simulink model "SystemComposer_Architecture"  (R2020a)
settings: Solver=VariableStepAuto  StartTime=0.0  StopTime=10.0  RelTol=1e-3
settings Model: Creator=pav4609  LastModifiedBy=pav4609

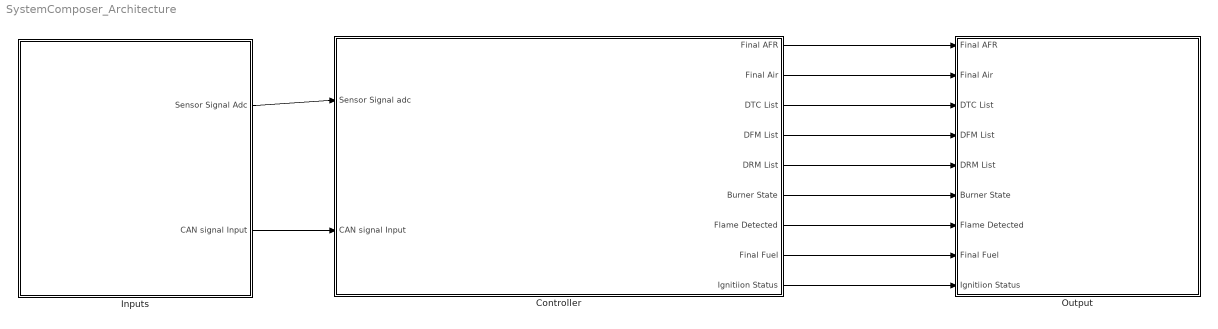
== system SystemComposer_Architecture ==
  Controller : Subsystem
      settings: PortSchema="{\"entries\":[{\"content\":{\"headerSize\":26,\"margin\":15,\"minimumSpacing\":25,\"sides\":[{\"content\":{\"connectorIds\":[\"In1\",\"In2\"]},\"type\":\"ConnectorPlacement.EquallySpacedRectSide\",\"uuid\":\"096bda3c-cb26-41de-ada6-ed8c82f4dc3e\"},{\"content\":{\"connectorIds\":[\"Out1\",\"Out2\",\"Out3\",\"Out4\",\"Out5\",\"Out6\",\"Out7\",\"Out8\",\"Out9\"],\"side\":\"RIGHT\"},\"type\":\"ConnectorPlacement.EquallySpacedRectSide\",\"uuid\":\"33a8afe9-c0b7-4d1e-b92f-6038b85d7ed2\"},{\"content\":{\"connectorIds\":[],\"side\":\"TOP\"},\"type\":\"ConnectorPlacement.EquallySpacedRectSide\",\"uuid\":\"f728da00-d767-486c-a498-31860175d68d\"}]},\"type\":\"ConnectorPlacement.EquallySpacedConnector\",\"uuid\":\"b1077154-7336-4249-93d2-0c64e27b627c\"}],\"packageUris\":[\"http://schema.mathworks.com/mf0/Connector/19700101\"],\"version\":\"1.0\"}"
  Inputs : Subsystem
      settings: PortSchema="{\"entries\":[{\"content\":{\"headerSize\":26,\"margin\":15,\"minimumSpacing\":25,\"sides\":[{\"content\":{\"connectorIds\":[]},\"type\":\"ConnectorPlacement.EquallySpacedRectSide\",\"uuid\":\"096bda3c-cb26-41de-ada6-ed8c82f4dc3e\"},{\"content\":{\"connectorIds\":[\"Out1\",\"Out2\"],\"side\":\"RIGHT\"},\"type\":\"ConnectorPlacement.EquallySpacedRectSide\",\"uuid\":\"33a8afe9-c0b7-4d1e-b92f-6038b85d7ed2\"},{\"content\":{\"connectorIds\":[],\"side\":\"TOP\"},\"type\":\"ConnectorPlacement.EquallySpacedRectSide\",\"uuid\":\"f728da00-d767-486c-a498-31860175d68d\"}]},\"type\":\"ConnectorPlacement.EquallySpacedConnector\",\"uuid\":\"b1077154-7336-4249-93d2-0c64e27b627c\"}],\"packageUris\":[\"http://schema.mathworks.com/mf0/Connector/19700101\"],\"version\":\"1.0\"}"
  Output : Subsystem
      settings: PortSchema="{\"entries\":[{\"content\":{\"headerSize\":26,\"margin\":15,\"minimumSpacing\":25,\"sides\":[{\"content\":{\"connectorIds\":[\"In3\",\"In4\",\"In5\",\"In6\",\"In7\",\"In8\",\"In9\",\"In1\",\"In2\"]},\"type\":\"ConnectorPlacement.EquallySpacedRectSide\",\"uuid\":\"096bda3c-cb26-41de-ada6-ed8c82f4dc3e\"},{\"content\":{\"connectorIds\":[],\"side\":\"RIGHT\"},\"type\":\"ConnectorPlacement.EquallySpacedRectSide\",\"uuid\":\"33a8afe9-c0b7-4d1e-b92f-6038b85d7ed2\"},{\"content\":{\"connectorIds\":[],\"side\":\"TOP\"},\"type\":\"ConnectorPlacement.EquallySpacedRectSide\",\"uuid\":\"f728da00-d767-486c-a498-31860175d68d\"},{\"content\":{\"connectorIds\":[],\"side\":\"BOTTOM\"},\"type\":\"ConnectorPlacement.EquallySpacedRectSide\",\"uuid\":\"2b26c1e7-6ba1-4f96-9e0c-c596cf4da347\"}]},\"type\":\"ConnectorPlacement.EquallySpacedConnector\",\"uuid\":\"b1077154-7336-4249-93d2-0c64e27b627c\"}],\"packageUris\":[\"http://schema.mathworks.com/mf0/Connector/19700101\"],\"version\":\"1.0\"}"
  wires:
  Inputs/1(Sensor Signal Adc) -> Controller/1(Sensor Signal adc)
  Inputs/2(CAN signal Input) -> Controller/2(CAN signal Input)
  Controller/1(Final AFR) -> Output/3(Final AFR)
  Controller/2(Final Air) -> Output/4(Final Air)
  Controller/3(DTC List) -> Output/5(DTC List)
  Controller/4(DFM List) -> Output/6(DFM List)
  Controller/5(DRM List) -> Output/7(DRM List)
  Controller/6(Burner State) -> Output/8(Burner State)
  Controller/7(Flame Detected) -> Output/9(Flame Detected)
  Controller/8(Final Fuel) -> Output/1(Final Fuel)
  Controller/9(Ignitiion Status) -> Output/2(Ignitiion Status)

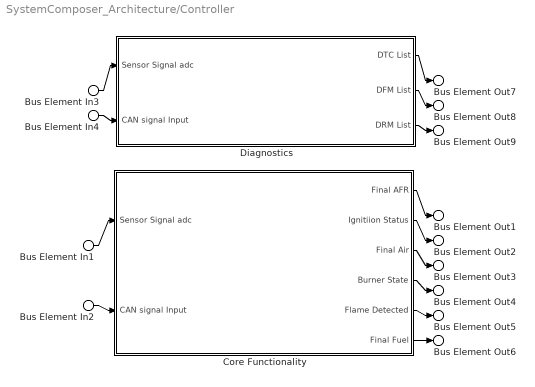
== system SystemComposer_Architecture/Controller ==
  Bus Element In1 : Inport  PortName=Sensor Signal adc
  Bus Element In3 : Inport  PortName=Sensor Signal adc
  Bus Element In2 : Inport  Port=2  PortName=CAN signal Input
  Bus Element In4 : Inport  Port=2  PortName=CAN signal Input
  Core Functionality : Subsystem
      settings: PortSchema="{\"entries\":[{\"content\":{\"headerSize\":26,\"margin\":15,\"minimumSpacing\":25,\"sides\":[{\"content\":{\"connectorIds\":[\"In1\",\"In2\"]},\"type\":\"ConnectorPlacement.EquallySpacedRectSide\",\"uuid\":\"096bda3c-cb26-41de-ada6-ed8c82f4dc3e\"},{\"content\":{\"connectorIds\":[\"Out1\",\"Out2\",\"Out3\",\"Out4\",\"Out5\",\"Out6\"],\"side\":\"RIGHT\"},\"type\":\"ConnectorPlacement.EquallySpacedRectSide\",\"uuid\":\"33a8afe9-c0b7-4d1e-b92f-6038b85d7ed2\"},{\"content\":{\"connectorIds\":[],\"side\":\"TOP\"},\"type\":\"ConnectorPlacement.EquallySpacedRectSide\",\"uuid\":\"f728da00-d767-486c-a498-31860175d68d\"}]},\"type\":\"ConnectorPlacement.EquallySpacedConnector\",\"uuid\":\"b1077154-7336-4249-93d2-0c64e27b627c\"}],\"packageUris\":[\"http://schema.mathworks.com/mf0/Connector/19700101\"],\"version\":\"1.0\"}"
  Diagnostics : Subsystem
      settings: PortSchema="{\"entries\":[{\"content\":{\"headerSize\":26,\"margin\":15,\"minimumSpacing\":25,\"sides\":[{\"content\":{\"connectorIds\":[\"In1\",\"In2\"]},\"type\":\"ConnectorPlacement.EquallySpacedRectSide\",\"uuid\":\"096bda3c-cb26-41de-ada6-ed8c82f4dc3e\"},{\"content\":{\"connectorIds\":[\"Out1\",\"Out2\",\"Out3\"],\"side\":\"RIGHT\"},\"type\":\"ConnectorPlacement.EquallySpacedRectSide\",\"uuid\":\"33a8afe9-c0b7-4d1e-b92f-6038b85d7ed2\"},{\"content\":{\"connectorIds\":[],\"side\":\"TOP\"},\"type\":\"ConnectorPlacement.EquallySpacedRectSide\",\"uuid\":\"f728da00-d767-486c-a498-31860175d68d\"}]},\"type\":\"ConnectorPlacement.EquallySpacedConnector\",\"uuid\":\"b1077154-7336-4249-93d2-0c64e27b627c\"}],\"packageUris\":[\"http://schema.mathworks.com/mf0/Connector/19700101\"],\"version\":\"1.0\"}"
  Bus Element Out1 : Outport  PortName=Final AFR
  Bus Element Out3 : Outport  Port=2  PortName=Final Air
  Bus Element Out7 : Outport  Port=3  PortName=DTC List
  Bus Element Out8 : Outport  Port=4  PortName=DFM List
  Bus Element Out9 : Outport  Port=5  PortName=DRM List
  Bus Element Out4 : Outport  Port=6  PortName=Burner State
  Bus Element Out5 : Outport  Port=7  PortName=Flame Detected
  Bus Element Out6 : Outport  Port=8  PortName=Final Fuel
  Bus Element Out2 : Outport  Port=9  PortName=Ignitiion Status
  wires:
  Bus Element In1/1 -> Core Functionality/1(Sensor Signal adc)
  Bus Element In2/1 -> Core Functionality/2(CAN signal Input)
  Bus Element In3/1 -> Diagnostics/1(Sensor Signal adc)
  Bus Element In4/1 -> Diagnostics/2(CAN signal Input)
  Core Functionality/1(Final AFR) -> Bus Element Out1/1
  Core Functionality/2(Ignitiion Status) -> Bus Element Out2/1
  Core Functionality/3(Final Air) -> Bus Element Out3/1
  Core Functionality/4(Burner State) -> Bus Element Out4/1
  Core Functionality/5(Flame Detected) -> Bus Element Out5/1
  Core Functionality/6(Final Fuel) -> Bus Element Out6/1
  Diagnostics/1(DTC List) -> Bus Element Out7/1
  Diagnostics/2(DFM List) -> Bus Element Out8/1
  Diagnostics/3(DRM List) -> Bus Element Out9/1

== system SystemComposer_Architecture/Inputs ==
  CAN : Subsystem
      settings: PortSchema="{\"entries\":[{\"content\":{\"headerSize\":26,\"margin\":15,\"minimumSpacing\":25,\"sides\":[{\"content\":{\"connectorIds\":[]},\"type\":\"ConnectorPlacement.EquallySpacedRectSide\",\"uuid\":\"096bda3c-cb26-41de-ada6-ed8c82f4dc3e\"},{\"content\":{\"connectorIds\":[\"Out1\"],\"side\":\"RIGHT\"},\"type\":\"ConnectorPlacement.EquallySpacedRectSide\",\"uuid\":\"33a8afe9-c0b7-4d1e-b92f-6038b85d7ed2\"},{\"content\":{\"connectorIds\":[],\"side\":\"TOP\"},\"type\":\"ConnectorPlacement.EquallySpacedRectSide\",\"uuid\":\"f728da00-d767-486c-a498-31860175d68d\"}]},\"type\":\"ConnectorPlacement.EquallySpacedConnector\",\"uuid\":\"b1077154-7336-4249-93d2-0c64e27b627c\"}],\"packageUris\":[\"http://schema.mathworks.com/mf0/Connector/19700101\"],\"version\":\"1.0\"}"
  Sensors : Subsystem
      settings: PortSchema="{\"entries\":[{\"content\":{\"headerSize\":26,\"margin\":15,\"minimumSpacing\":25,\"sides\":[{\"content\":{\"connectorIds\":[]},\"type\":\"ConnectorPlacement.EquallySpacedRectSide\",\"uuid\":\"096bda3c-cb26-41de-ada6-ed8c82f4dc3e\"},{\"content\":{\"connectorIds\":[\"Out1\"],\"side\":\"RIGHT\"},\"type\":\"ConnectorPlacement.EquallySpacedRectSide\",\"uuid\":\"33a8afe9-c0b7-4d1e-b92f-6038b85d7ed2\"},{\"content\":{\"connectorIds\":[],\"side\":\"TOP\"},\"type\":\"ConnectorPlacement.EquallySpacedRectSide\",\"uuid\":\"f728da00-d767-486c-a498-31860175d68d\"}]},\"type\":\"ConnectorPlacement.EquallySpacedConnector\",\"uuid\":\"b1077154-7336-4249-93d2-0c64e27b627c\"}],\"packageUris\":[\"http://schema.mathworks.com/mf0/Connector/19700101\"],\"version\":\"1.0\"}"
  Bus Element Out1 : Outport  PortName=Sensor Signal Adc
  Bus Element Out2 : Outport  Port=2  PortName=CAN signal Input
  wires:
  Sensors/1(Sensor Signal Adc) -> Bus Element Out1/1
  CAN/1(CAN signal Input) -> Bus Element Out2/1

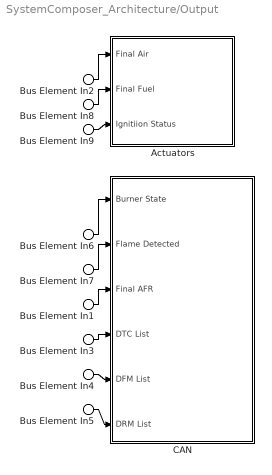
== system SystemComposer_Architecture/Output ==
  Bus Element In8 : Inport  PortName=Final Fuel
  Bus Element In9 : Inport  Port=2  PortName=Ignitiion Status
  Bus Element In1 : Inport  Port=3  PortName=Final AFR
  Bus Element In2 : Inport  Port=4  PortName=Final Air
  Bus Element In3 : Inport  Port=5  PortName=DTC List
  Bus Element In4 : Inport  Port=6  PortName=DFM List
  Bus Element In5 : Inport  Port=7  PortName=DRM List
  Bus Element In6 : Inport  Port=8  PortName=Burner State
  Bus Element In7 : Inport  Port=9  PortName=Flame Detected
  Actuators : Subsystem
      settings: PortSchema="{\"entries\":[{\"content\":{\"headerSize\":26,\"margin\":15,\"minimumSpacing\":25,\"sides\":[{\"content\":{\"connectorIds\":[\"In1\",\"In2\",\"In3\"]},\"type\":\"ConnectorPlacement.EquallySpacedRectSide\",\"uuid\":\"096bda3c-cb26-41de-ada6-ed8c82f4dc3e\"},{\"content\":{\"connectorIds\":[],\"side\":\"RIGHT\"},\"type\":\"ConnectorPlacement.EquallySpacedRectSide\",\"uuid\":\"33a8afe9-c0b7-4d1e-b92f-6038b85d7ed2\"},{\"content\":{\"connectorIds\":[],\"side\":\"TOP\"},\"type\":\"ConnectorPlacement.EquallySpacedRectSide\",\"uuid\":\"f728da00-d767-486c-a498-31860175d68d\"}]},\"type\":\"ConnectorPlacement.EquallySpacedConnector\",\"uuid\":\"b1077154-7336-4249-93d2-0c64e27b627c\"}],\"packageUris\":[\"http://schema.mathworks.com/mf0/Connector/19700101\"],\"version\":\"1.0\"}"
  CAN : Subsystem
      settings: PortSchema="{\"entries\":[{\"content\":{\"headerSize\":26,\"margin\":15,\"minimumSpacing\":25,\"sides\":[{\"content\":{\"connectorIds\":[\"In1\",\"In2\",\"In3\",\"In4\",\"In5\",\"In6\"]},\"type\":\"ConnectorPlacement.EquallySpacedRectSide\",\"uuid\":\"096bda3c-cb26-41de-ada6-ed8c82f4dc3e\"},{\"content\":{\"connectorIds\":[],\"side\":\"RIGHT\"},\"type\":\"ConnectorPlacement.EquallySpacedRectSide\",\"uuid\":\"33a8afe9-c0b7-4d1e-b92f-6038b85d7ed2\"},{\"content\":{\"connectorIds\":[],\"side\":\"TOP\"},\"type\":\"ConnectorPlacement.EquallySpacedRectSide\",\"uuid\":\"f728da00-d767-486c-a498-31860175d68d\"}]},\"type\":\"ConnectorPlacement.EquallySpacedConnector\",\"uuid\":\"b1077154-7336-4249-93d2-0c64e27b627c\"}],\"packageUris\":[\"http://schema.mathworks.com/mf0/Connector/19700101\"],\"version\":\"1.0\"}"
  wires:
  Bus Element In2/1 -> Actuators/1(Final Air)
  Bus Element In8/1 -> Actuators/2(Final Fuel)
  Bus Element In9/1 -> Actuators/3(Ignitiion Status)
  Bus Element In6/1 -> CAN/1(Burner State)
  Bus Element In7/1 -> CAN/2(Flame Detected)
  Bus Element In1/1 -> CAN/3(Final AFR)
  Bus Element In3/1 -> CAN/4(DTC List)
  Bus Element In4/1 -> CAN/5(DFM List)
  Bus Element In5/1 -> CAN/6(DRM List)

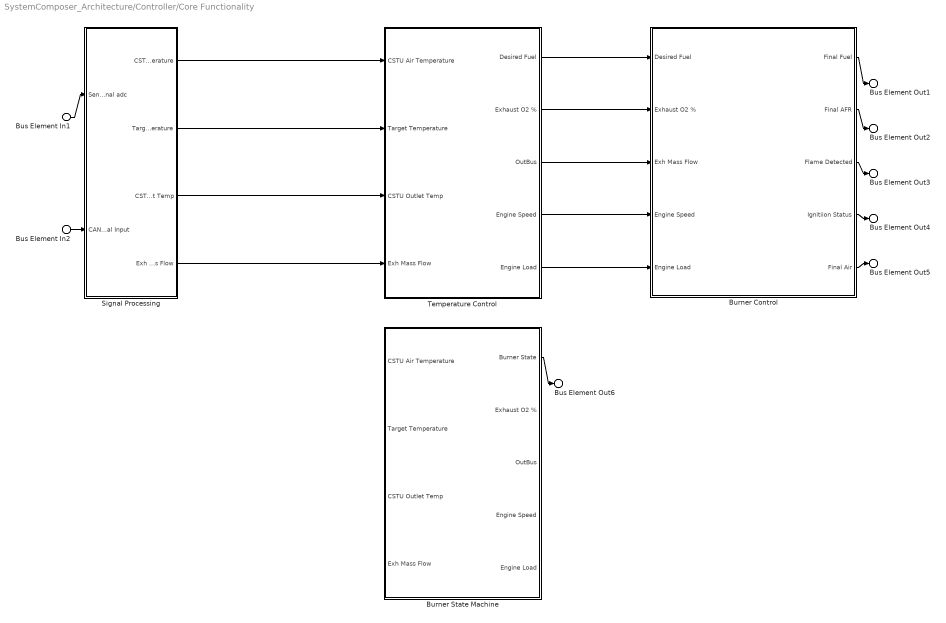
== system SystemComposer_Architecture/Controller/Core Functionality ==
  Bus Element In1 : Inport  PortName=Sensor Signal adc
  Bus Element In2 : Inport  Port=2  PortName=CAN signal Input
  Burner Control : Subsystem
      settings: PortSchema="{\"entries\":[{\"content\":{\"headerSize\":26,\"margin\":15,\"minimumSpacing\":25,\"sides\":[{\"content\":{\"connectorIds\":[\"In1\",\"In2\",\"In3\",\"In4\",\"In5\"]},\"type\":\"ConnectorPlacement.EquallySpacedRectSide\",\"uuid\":\"096bda3c-cb26-41de-ada6-ed8c82f4dc3e\"},{\"content\":{\"connectorIds\":[\"Out1\",\"Out2\",\"Out3\",\"Out4\",\"Out5\"],\"side\":\"RIGHT\"},\"type\":\"ConnectorPlacement.EquallySpacedRectSide\",\"uuid\":\"33a8afe9-c0b7-4d1e-b92f-6038b85d7ed2\"},{\"content\":{\"connectorIds\":[],\"side\":\"TOP\"},\"type\":\"ConnectorPlacement.EquallySpacedRectSide\",\"uuid\":\"f728da00-d767-486c-a498-31860175d68d\"}]},\"type\":\"ConnectorPlacement.EquallySpacedConnector\",\"uuid\":\"b1077154-7336-4249-93d2-0c64e27b627c\"}],\"packageUris\":[\"http://schema.mathworks.com/mf0/Connector/19700101\"],\"version\":\"1.0\"}"
  Burner State Machine : Subsystem
      settings: PortSchema="{\"entries\":[{\"content\":{\"headerSize\":26,\"margin\":15,\"minimumSpacing\":25,\"sides\":[{\"content\":{\"connectorIds\":[\"In1\",\"In2\",\"In3\",\"In4\"]},\"type\":\"ConnectorPlacement.EquallySpacedRectSide\",\"uuid\":\"096bda3c-cb26-41de-ada6-ed8c82f4dc3e\"},{\"content\":{\"connectorIds\":[\"Out1\",\"Out2\",\"Out3\",\"Out4\",\"Out5\"],\"side\":\"RIGHT\"},\"type\":\"ConnectorPlacement.EquallySpacedRectSide\",\"uuid\":\"33a8afe9-c0b7-4d1e-b92f-6038b85d7ed2\"},{\"content\":{\"connectorIds\":[],\"side\":\"TOP\"},\"type\":\"ConnectorPlacement.EquallySpacedRectSide\",\"uuid\":\"f728da00-d767-486c-a498-31860175d68d\"}]},\"type\":\"ConnectorPlacement.EquallySpacedConnector\",\"uuid\":\"b1077154-7336-4249-93d2-0c64e27b627c\"}],\"packageUris\":[\"http://schema.mathworks.com/mf0/Connector/19700101\"],\"version\":\"1.0\"}"
  Signal Processing : Subsystem
      settings: PortSchema="{\"entries\":[{\"content\":{\"headerSize\":26,\"margin\":15,\"minimumSpacing\":25,\"sides\":[{\"content\":{\"connectorIds\":[\"In1\",\"In2\"]},\"type\":\"ConnectorPlacement.EquallySpacedRectSide\",\"uuid\":\"096bda3c-cb26-41de-ada6-ed8c82f4dc3e\"},{\"content\":{\"connectorIds\":[\"Out1\",\"Out2\",\"Out3\",\"Out4\"],\"side\":\"RIGHT\"},\"type\":\"ConnectorPlacement.EquallySpacedRectSide\",\"uuid\":\"33a8afe9-c0b7-4d1e-b92f-6038b85d7ed2\"},{\"content\":{\"connectorIds\":[],\"side\":\"TOP\"},\"type\":\"ConnectorPlacement.EquallySpacedRectSide\",\"uuid\":\"f728da00-d767-486c-a498-31860175d68d\"}]},\"type\":\"ConnectorPlacement.EquallySpacedConnector\",\"uuid\":\"b1077154-7336-4249-93d2-0c64e27b627c\"}],\"packageUris\":[\"http://schema.mathworks.com/mf0/Connector/19700101\"],\"version\":\"1.0\"}"
  Temperature Control : Subsystem
      settings: PortSchema="{\"entries\":[{\"content\":{\"headerSize\":26,\"margin\":15,\"minimumSpacing\":25,\"sides\":[{\"content\":{\"connectorIds\":[\"In1\",\"In2\",\"In3\",\"In4\"]},\"type\":\"ConnectorPlacement.EquallySpacedRectSide\",\"uuid\":\"096bda3c-cb26-41de-ada6-ed8c82f4dc3e\"},{\"content\":{\"connectorIds\":[\"Out1\",\"Out2\",\"Out3\",\"Out4\",\"Out5\"],\"side\":\"RIGHT\"},\"type\":\"ConnectorPlacement.EquallySpacedRectSide\",\"uuid\":\"33a8afe9-c0b7-4d1e-b92f-6038b85d7ed2\"},{\"content\":{\"connectorIds\":[],\"side\":\"TOP\"},\"type\":\"ConnectorPlacement.EquallySpacedRectSide\",\"uuid\":\"f728da00-d767-486c-a498-31860175d68d\"}]},\"type\":\"ConnectorPlacement.EquallySpacedConnector\",\"uuid\":\"b1077154-7336-4249-93d2-0c64e27b627c\"}],\"packageUris\":[\"http://schema.mathworks.com/mf0/Connector/19700101\"],\"version\":\"1.0\"}"
  Bus Element Out2 : Outport  PortName=Final AFR
  Bus Element Out4 : Outport  Port=2  PortName=Ignitiion Status
  Bus Element Out5 : Outport  Port=3  PortName=Final Air
  Bus Element Out6 : Outport  Port=4  PortName=Burner State
  Bus Element Out3 : Outport  Port=5  PortName=Flame Detected
  Bus Element Out1 : Outport  Port=6  PortName=Final Fuel
  wires:
  Bus Element In1/1 -> Signal Processing/1(Sensor Signal adc)
  Bus Element In2/1 -> Signal Processing/2(CAN signal Input)
  Temperature Control/1(Desired Fuel) -> Burner Control/1(Desired Fuel)
  Temperature Control/2(Exhaust O2 %) -> Burner Control/2(Exhaust O2 %)
  Temperature Control/3(OutBus) -> Burner Control/3(Exh Mass Flow)
  Temperature Control/4(Engine Speed) -> Burner Control/4(Engine Speed)
  Temperature Control/5(Engine Load) -> Burner Control/5(Engine Load)
  Signal Processing/1(CSTU Air Temperature) -> Temperature Control/1(CSTU Air Temperature)
  Signal Processing/2(Target Temperature) -> Temperature Control/2(Target Temperature)
  Signal Processing/3(CSTU Outlet Temp) -> Temperature Control/3(CSTU Outlet Temp)
  Signal Processing/4(Exh Mass Flow) -> Temperature Control/4(Exh Mass Flow)
  Burner Control/1(Final Fuel) -> Bus Element Out1/1
  Burner Control/2(Final AFR) -> Bus Element Out2/1
  Burner Control/3(Flame Detected) -> Bus Element Out3/1
  Burner Control/4(Ignitiion Status) -> Bus Element Out4/1
  Burner Control/5(Final Air) -> Bus Element Out5/1
  Burner State Machine/1(Burner State) -> Bus Element Out6/1

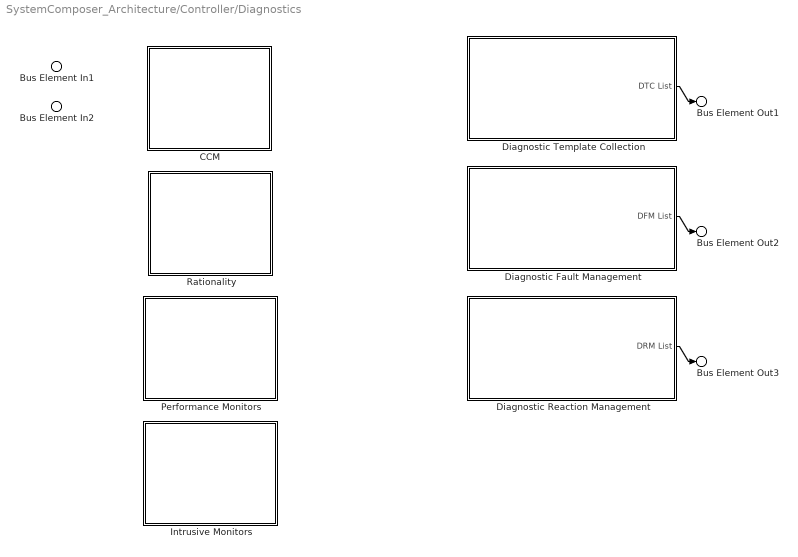
== system SystemComposer_Architecture/Controller/Diagnostics ==
  Bus Element In1 : Inport  PortName=Sensor Signal adc
  Bus Element In2 : Inport  Port=2  PortName=CAN signal Input
  CCM : Subsystem
      settings: PortSchema="{\"entries\":[{\"content\":{\"headerSize\":26,\"margin\":15,\"minimumSpacing\":25,\"sides\":[{\"content\":{\"connectorIds\":[]},\"type\":\"ConnectorPlacement.EquallySpacedRectSide\",\"uuid\":\"096bda3c-cb26-41de-ada6-ed8c82f4dc3e\"},{\"content\":{\"connectorIds\":[],\"side\":\"RIGHT\"},\"type\":\"ConnectorPlacement.EquallySpacedRectSide\",\"uuid\":\"33a8afe9-c0b7-4d1e-b92f-6038b85d7ed2\"},{\"content\":{\"connectorIds\":[],\"side\":\"TOP\"},\"type\":\"ConnectorPlacement.EquallySpacedRectSide\",\"uuid\":\"f728da00-d767-486c-a498-31860175d68d\"}]},\"type\":\"ConnectorPlacement.EquallySpacedConnector\",\"uuid\":\"b1077154-7336-4249-93d2-0c64e27b627c\"}],\"packageUris\":[\"http://schema.mathworks.com/mf0/Connector/19700101\"],\"version\":\"1.0\"}"
  Diagnostic Fault Management : Subsystem
      settings: PortSchema="{\"entries\":[{\"content\":{\"headerSize\":26,\"margin\":15,\"minimumSpacing\":25,\"sides\":[{\"content\":{\"connectorIds\":[]},\"type\":\"ConnectorPlacement.EquallySpacedRectSide\",\"uuid\":\"096bda3c-cb26-41de-ada6-ed8c82f4dc3e\"},{\"content\":{\"connectorIds\":[\"Out1\"],\"side\":\"RIGHT\"},\"type\":\"ConnectorPlacement.EquallySpacedRectSide\",\"uuid\":\"33a8afe9-c0b7-4d1e-b92f-6038b85d7ed2\"},{\"content\":{\"connectorIds\":[],\"side\":\"TOP\"},\"type\":\"ConnectorPlacement.EquallySpacedRectSide\",\"uuid\":\"f728da00-d767-486c-a498-31860175d68d\"}]},\"type\":\"ConnectorPlacement.EquallySpacedConnector\",\"uuid\":\"b1077154-7336-4249-93d2-0c64e27b627c\"}],\"packageUris\":[\"http://schema.mathworks.com/mf0/Connector/19700101\"],\"version\":\"1.0\"}"
  Diagnostic Reaction Management : Subsystem
      settings: PortSchema="{\"entries\":[{\"content\":{\"headerSize\":26,\"margin\":15,\"minimumSpacing\":25,\"sides\":[{\"content\":{\"connectorIds\":[]},\"type\":\"ConnectorPlacement.EquallySpacedRectSide\",\"uuid\":\"096bda3c-cb26-41de-ada6-ed8c82f4dc3e\"},{\"content\":{\"connectorIds\":[\"Out1\"],\"side\":\"RIGHT\"},\"type\":\"ConnectorPlacement.EquallySpacedRectSide\",\"uuid\":\"33a8afe9-c0b7-4d1e-b92f-6038b85d7ed2\"},{\"content\":{\"connectorIds\":[],\"side\":\"TOP\"},\"type\":\"ConnectorPlacement.EquallySpacedRectSide\",\"uuid\":\"f728da00-d767-486c-a498-31860175d68d\"}]},\"type\":\"ConnectorPlacement.EquallySpacedConnector\",\"uuid\":\"b1077154-7336-4249-93d2-0c64e27b627c\"}],\"packageUris\":[\"http://schema.mathworks.com/mf0/Connector/19700101\"],\"version\":\"1.0\"}"
  Diagnostic Template Collection : Subsystem
      settings: PortSchema="{\"entries\":[{\"content\":{\"headerSize\":26,\"margin\":15,\"minimumSpacing\":25,\"sides\":[{\"content\":{\"connectorIds\":[]},\"type\":\"ConnectorPlacement.EquallySpacedRectSide\",\"uuid\":\"096bda3c-cb26-41de-ada6-ed8c82f4dc3e\"},{\"content\":{\"connectorIds\":[\"Out1\"],\"side\":\"RIGHT\"},\"type\":\"ConnectorPlacement.EquallySpacedRectSide\",\"uuid\":\"33a8afe9-c0b7-4d1e-b92f-6038b85d7ed2\"},{\"content\":{\"connectorIds\":[],\"side\":\"TOP\"},\"type\":\"ConnectorPlacement.EquallySpacedRectSide\",\"uuid\":\"f728da00-d767-486c-a498-31860175d68d\"}]},\"type\":\"ConnectorPlacement.EquallySpacedConnector\",\"uuid\":\"b1077154-7336-4249-93d2-0c64e27b627c\"}],\"packageUris\":[\"http://schema.mathworks.com/mf0/Connector/19700101\"],\"version\":\"1.0\"}"
  Intrusive Monitors : Subsystem
      settings: PortSchema="{\"entries\":[{\"content\":{\"headerSize\":26,\"margin\":15,\"minimumSpacing\":25,\"sides\":[{\"content\":{\"connectorIds\":[]},\"type\":\"ConnectorPlacement.EquallySpacedRectSide\",\"uuid\":\"096bda3c-cb26-41de-ada6-ed8c82f4dc3e\"},{\"content\":{\"connectorIds\":[],\"side\":\"RIGHT\"},\"type\":\"ConnectorPlacement.EquallySpacedRectSide\",\"uuid\":\"33a8afe9-c0b7-4d1e-b92f-6038b85d7ed2\"},{\"content\":{\"connectorIds\":[],\"side\":\"TOP\"},\"type\":\"ConnectorPlacement.EquallySpacedRectSide\",\"uuid\":\"f728da00-d767-486c-a498-31860175d68d\"}]},\"type\":\"ConnectorPlacement.EquallySpacedConnector\",\"uuid\":\"b1077154-7336-4249-93d2-0c64e27b627c\"}],\"packageUris\":[\"http://schema.mathworks.com/mf0/Connector/19700101\"],\"version\":\"1.0\"}"
  Performance Monitors : Subsystem
      settings: PortSchema="{\"entries\":[{\"content\":{\"headerSize\":26,\"margin\":15,\"minimumSpacing\":25,\"sides\":[{\"content\":{\"connectorIds\":[]},\"type\":\"ConnectorPlacement.EquallySpacedRectSide\",\"uuid\":\"096bda3c-cb26-41de-ada6-ed8c82f4dc3e\"},{\"content\":{\"connectorIds\":[],\"side\":\"RIGHT\"},\"type\":\"ConnectorPlacement.EquallySpacedRectSide\",\"uuid\":\"33a8afe9-c0b7-4d1e-b92f-6038b85d7ed2\"},{\"content\":{\"connectorIds\":[],\"side\":\"TOP\"},\"type\":\"ConnectorPlacement.EquallySpacedRectSide\",\"uuid\":\"f728da00-d767-486c-a498-31860175d68d\"}]},\"type\":\"ConnectorPlacement.EquallySpacedConnector\",\"uuid\":\"b1077154-7336-4249-93d2-0c64e27b627c\"}],\"packageUris\":[\"http://schema.mathworks.com/mf0/Connector/19700101\"],\"version\":\"1.0\"}"
  Rationality : Subsystem
      settings: PortSchema="{\"entries\":[{\"content\":{\"headerSize\":26,\"margin\":15,\"minimumSpacing\":25,\"sides\":[{\"content\":{\"connectorIds\":[]},\"type\":\"ConnectorPlacement.EquallySpacedRectSide\",\"uuid\":\"096bda3c-cb26-41de-ada6-ed8c82f4dc3e\"},{\"content\":{\"connectorIds\":[],\"side\":\"RIGHT\"},\"type\":\"ConnectorPlacement.EquallySpacedRectSide\",\"uuid\":\"33a8afe9-c0b7-4d1e-b92f-6038b85d7ed2\"},{\"content\":{\"connectorIds\":[],\"side\":\"TOP\"},\"type\":\"ConnectorPlacement.EquallySpacedRectSide\",\"uuid\":\"f728da00-d767-486c-a498-31860175d68d\"}]},\"type\":\"ConnectorPlacement.EquallySpacedConnector\",\"uuid\":\"b1077154-7336-4249-93d2-0c64e27b627c\"}],\"packageUris\":[\"http://schema.mathworks.com/mf0/Connector/19700101\"],\"version\":\"1.0\"}"
  Bus Element Out1 : Outport  PortName=DTC List
  Bus Element Out2 : Outport  Port=2  PortName=DFM List
  Bus Element Out3 : Outport  Port=3  PortName=DRM List
  wires:
  Diagnostic Template Collection/1(DTC List) -> Bus Element Out1/1
  Diagnostic Fault Management/1(DFM List) -> Bus Element Out2/1
  Diagnostic Reaction Management/1(DRM List) -> Bus Element Out3/1

== system SystemComposer_Architecture/Inputs/CAN ==
  Bus Element Out1 : Outport  PortName=CAN signal Input

== system SystemComposer_Architecture/Inputs/Sensors ==
  Bus Element Out1 : Outport  PortName=Sensor Signal Adc

== system SystemComposer_Architecture/Output/Actuators ==
  Bus Element In1 : Inport  PortName=Final Air
  Bus Element In2 : Inport  Port=2  PortName=Final Fuel
  Bus Element In3 : Inport  Port=3  PortName=Ignitiion Status

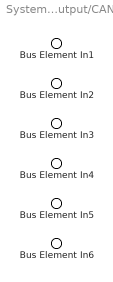
== system SystemComposer_Architecture/Output/CAN ==
  Bus Element In1 : Inport  PortName=Burner State
  Bus Element In2 : Inport  Port=2  PortName=Flame Detected
  Bus Element In3 : Inport  Port=3  PortName=Final AFR
  Bus Element In4 : Inport  Port=4  PortName=DTC List
  Bus Element In5 : Inport  Port=5  PortName=DFM List
  Bus Element In6 : Inport  Port=6  PortName=DRM List

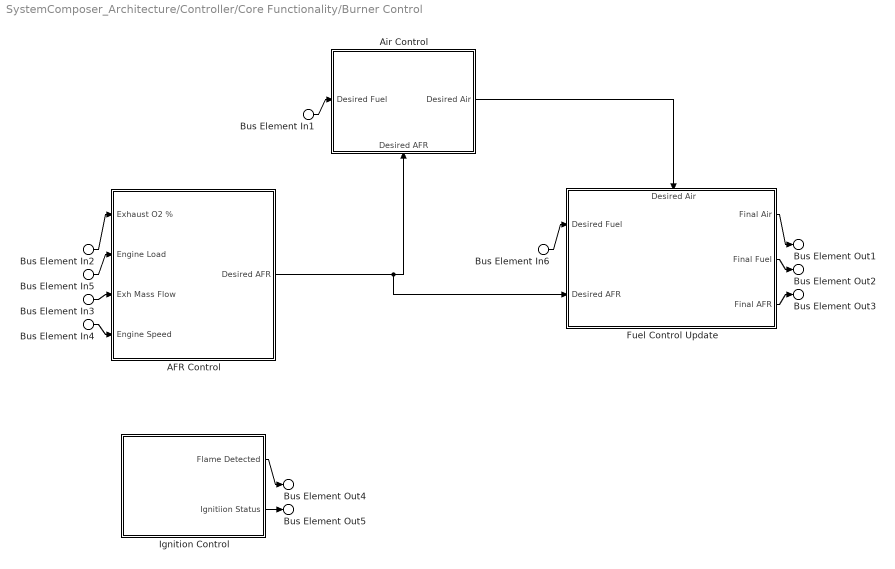
== system SystemComposer_Architecture/Controller/Core Functionality/Burner Control ==
  Bus Element In1 : Inport  PortName=Desired Fuel
  Bus Element In6 : Inport  PortName=Desired Fuel
  Bus Element In2 : Inport  Port=2  PortName=Exhaust O2 %
  Bus Element In3 : Inport  Port=3  PortName=Exh Mass Flow
  Bus Element In4 : Inport  Port=4  PortName=Engine Speed
  Bus Element In5 : Inport  Port=5  PortName=Engine Load
  AFR Control : Subsystem
      settings: PortSchema="{\"entries\":[{\"content\":{\"headerSize\":26,\"margin\":15,\"minimumSpacing\":25,\"sides\":[{\"content\":{\"connectorIds\":[\"In3\",\"In2\",\"In4\",\"In1\"]},\"type\":\"ConnectorPlacement.EquallySpacedRectSide\",\"uuid\":\"096bda3c-cb26-41de-ada6-ed8c82f4dc3e\"},{\"content\":{\"connectorIds\":[\"Out1\"],\"side\":\"RIGHT\"},\"type\":\"ConnectorPlacement.EquallySpacedRectSide\",\"uuid\":\"33a8afe9-c0b7-4d1e-b92f-6038b85d7ed2\"},{\"content\":{\"connectorIds\":[],\"side\":\"TOP\"},\"type\":\"ConnectorPlacement.EquallySpacedRectSide\",\"uuid\":\"f728da00-d767-486c-a498-31860175d68d\"},{\"content\":{\"connectorIds\":[],\"side\":\"BOTTOM\"},\"type\":\"ConnectorPlacement.EquallySpacedRectSide\",\"uuid\":\"dc244666-318a-4643-9e94-467c3bf88959\"}]},\"type\":\"ConnectorPlacement.EquallySpacedConnector\",\"uuid\":\"b1077154-7336-4249-93d2-0c64e27b627c\"}],\"packageUris\":[\"http://schema.mathworks.com/mf0/Connector/19700101\"],\"version\":\"1.0\"}"
  Air Control : Subsystem
      settings: PortSchema="{\"entries\":[{\"content\":{\"headerSize\":26,\"margin\":15,\"minimumSpacing\":25,\"sides\":[{\"content\":{\"connectorIds\":[\"In2\"]},\"type\":\"ConnectorPlacement.EquallySpacedRectSide\",\"uuid\":\"096bda3c-cb26-41de-ada6-ed8c82f4dc3e\"},{\"content\":{\"connectorIds\":[\"Out1\"],\"side\":\"RIGHT\"},\"type\":\"ConnectorPlacement.EquallySpacedRectSide\",\"uuid\":\"33a8afe9-c0b7-4d1e-b92f-6038b85d7ed2\"},{\"content\":{\"connectorIds\":[],\"side\":\"TOP\"},\"type\":\"ConnectorPlacement.EquallySpacedRectSide\",\"uuid\":\"f728da00-d767-486c-a498-31860175d68d\"},{\"content\":{\"connectorIds\":[\"In1\"],\"side\":\"BOTTOM\"},\"type\":\"ConnectorPlacement.EquallySpacedRectSide\",\"uuid\":\"82f04bf9-f10d-4aad-bb32-e7ee3f14b728\"}]},\"type\":\"ConnectorPlacement.EquallySpacedConnector\",\"uuid\":\"b1077154-7336-4249-93d2-0c64e27b627c\"}],\"packageUris\":[\"http://schema.mathworks.com/mf0/Connector/19700101\"],\"version\":\"1.0\"}"
  Fuel Control Update : Subsystem
      settings: PortSchema="{\"entries\":[{\"content\":{\"headerSize\":26,\"margin\":15,\"minimumSpacing\":25,\"sides\":[{\"content\":{\"connectorIds\":[\"In1\",\"In2\"]},\"type\":\"ConnectorPlacement.EquallySpacedRectSide\",\"uuid\":\"096bda3c-cb26-41de-ada6-ed8c82f4dc3e\"},{\"content\":{\"connectorIds\":[\"Out1\",\"Out2\",\"Out3\"],\"side\":\"RIGHT\"},\"type\":\"ConnectorPlacement.EquallySpacedRectSide\",\"uuid\":\"33a8afe9-c0b7-4d1e-b92f-6038b85d7ed2\"},{\"content\":{\"connectorIds\":[\"In3\"],\"side\":\"TOP\"},\"type\":\"ConnectorPlacement.EquallySpacedRectSide\",\"uuid\":\"f728da00-d767-486c-a498-31860175d68d\"}]},\"type\":\"ConnectorPlacement.EquallySpacedConnector\",\"uuid\":\"b1077154-7336-4249-93d2-0c64e27b627c\"}],\"packageUris\":[\"http://schema.mathworks.com/mf0/Connector/19700101\"],\"version\":\"1.0\"}"
  Ignition Control : Subsystem
      settings: PortSchema="{\"entries\":[{\"content\":{\"headerSize\":26,\"margin\":15,\"minimumSpacing\":25,\"sides\":[{\"content\":{\"connectorIds\":[]},\"type\":\"ConnectorPlacement.EquallySpacedRectSide\",\"uuid\":\"096bda3c-cb26-41de-ada6-ed8c82f4dc3e\"},{\"content\":{\"connectorIds\":[\"Out1\",\"Out2\"],\"side\":\"RIGHT\"},\"type\":\"ConnectorPlacement.EquallySpacedRectSide\",\"uuid\":\"33a8afe9-c0b7-4d1e-b92f-6038b85d7ed2\"},{\"content\":{\"connectorIds\":[],\"side\":\"TOP\"},\"type\":\"ConnectorPlacement.EquallySpacedRectSide\",\"uuid\":\"f728da00-d767-486c-a498-31860175d68d\"}]},\"type\":\"ConnectorPlacement.EquallySpacedConnector\",\"uuid\":\"b1077154-7336-4249-93d2-0c64e27b627c\"}],\"packageUris\":[\"http://schema.mathworks.com/mf0/Connector/19700101\"],\"version\":\"1.0\"}"
  Bus Element Out2 : Outport  PortName=Final Fuel
  Bus Element Out3 : Outport  Port=2  PortName=Final AFR
  Bus Element Out4 : Outport  Port=3  PortName=Flame Detected
  Bus Element Out5 : Outport  Port=4  PortName=Ignitiion Status
  Bus Element Out1 : Outport  Port=5  PortName=Final Air
  wires:
  Bus Element In1/1 -> Air Control/2(Desired Fuel)
  Bus Element In2/1 -> AFR Control/3(Exhaust O2 %)
  Bus Element In3/1 -> AFR Control/4(Exh Mass Flow)
  Bus Element In4/1 -> AFR Control/1(Engine Speed)
  Bus Element In5/1 -> AFR Control/2(Engine Load)
  Air Control/1(Desired Air) -> Fuel Control Update/3(Desired Air)
  AFR Control/1(Desired AFR) -> Fuel Control Update/2(Desired AFR), Air Control/1(Desired AFR)
  Bus Element In6/1 -> Fuel Control Update/1(Desired Fuel)
  Fuel Control Update/1(Final Air) -> Bus Element Out1/1
  Fuel Control Update/2(Final Fuel) -> Bus Element Out2/1
  Fuel Control Update/3(Final AFR) -> Bus Element Out3/1
  Ignition Control/1(Flame Detected) -> Bus Element Out4/1
  Ignition Control/2(Ignitiion Status) -> Bus Element Out5/1

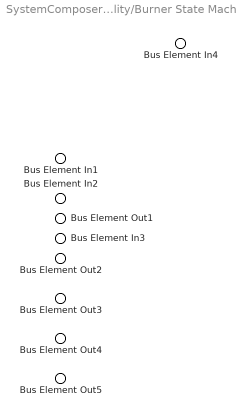
== system SystemComposer_Architecture/Controller/Core Functionality/Burner State Machine ==
  Bus Element In4 : Inport  PortName=CSTU Air Temperature
  Bus Element In1 : Inport  Port=2  PortName=Target Temperature
  Bus Element In2 : Inport  Port=3  PortName=CSTU Outlet Temp
  Bus Element In3 : Inport  Port=4  PortName=Exh Mass Flow
  Bus Element Out1 : Outport  PortName=Burner State
  Bus Element Out2 : Outport  Port=2  PortName=Exhaust O2 %
  Bus Element Out3 : Outport  Port=3  PortName=OutBus
  Bus Element Out4 : Outport  Port=4  PortName=Engine Speed
  Bus Element Out5 : Outport  Port=5  PortName=Engine Load

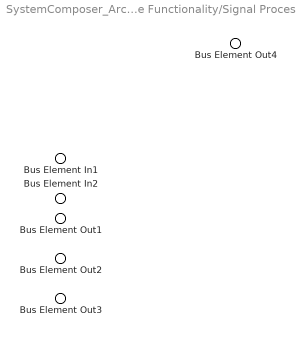
== system SystemComposer_Architecture/Controller/Core Functionality/Signal Processing ==
  Bus Element In1 : Inport  PortName=Sensor Signal adc
  Bus Element In2 : Inport  Port=2  PortName=CAN signal Input
  Bus Element Out4 : Outport  PortName=CSTU Air Temperature
  Bus Element Out1 : Outport  Port=2  PortName=Target Temperature
  Bus Element Out2 : Outport  Port=3  PortName=CSTU Outlet Temp
  Bus Element Out3 : Outport  Port=4  PortName=Exh Mass Flow

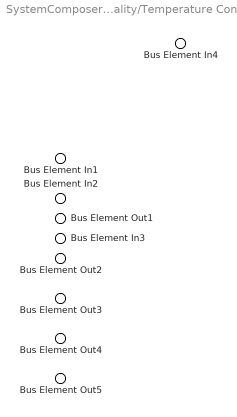
== system SystemComposer_Architecture/Controller/Core Functionality/Temperature Control ==
  Bus Element In4 : Inport  PortName=CSTU Air Temperature
  Bus Element In1 : Inport  Port=2  PortName=Target Temperature
  Bus Element In2 : Inport  Port=3  PortName=CSTU Outlet Temp
  Bus Element In3 : Inport  Port=4  PortName=Exh Mass Flow
  Bus Element Out1 : Outport  PortName=Desired Fuel
  Bus Element Out2 : Outport  Port=2  PortName=Exhaust O2 %
  Bus Element Out3 : Outport  Port=3  PortName=OutBus
  Bus Element Out4 : Outport  Port=4  PortName=Engine Speed
  Bus Element Out5 : Outport  Port=5  PortName=Engine Load

== system SystemComposer_Architecture/Controller/Diagnostics/CCM ==

== system SystemComposer_Architecture/Controller/Diagnostics/Diagnostic Fault Management ==
  Bus Element Out1 : Outport  PortName=DFM List

== system SystemComposer_Architecture/Controller/Diagnostics/Diagnostic Reaction Management ==
  Bus Element Out1 : Outport  PortName=DRM List

== system SystemComposer_Architecture/Controller/Diagnostics/Diagnostic Template Collection ==
  Bus Element Out1 : Outport  PortName=DTC List

== system SystemComposer_Architecture/Controller/Diagnostics/Intrusive Monitors ==

== system SystemComposer_Architecture/Controller/Diagnostics/Performance Monitors ==

== system SystemComposer_Architecture/Controller/Diagnostics/Rationality ==

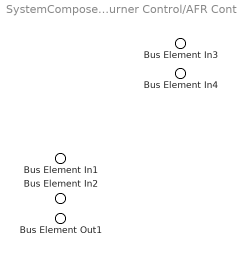
== system SystemComposer_Architecture/Controller/Core Functionality/Burner Control/AFR Control ==
  Bus Element In3 : Inport  PortName=Engine Speed
  Bus Element In4 : Inport  Port=2  PortName=Engine Load
  Bus Element In1 : Inport  Port=3  PortName=Exhaust O2 %
  Bus Element In2 : Inport  Port=4  PortName=Exh Mass Flow
  Bus Element Out1 : Outport  PortName=Desired AFR

== system SystemComposer_Architecture/Controller/Core Functionality/Burner Control/Air Control ==
  Bus Element In2 : Inport  PortName=Desired AFR
  Bus Element In1 : Inport  Port=2  PortName=Desired Fuel
  Bus Element Out1 : Outport  PortName=Desired Air

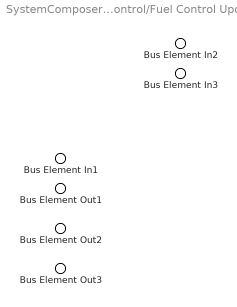
== system SystemComposer_Architecture/Controller/Core Functionality/Burner Control/Fuel Control Update ==
  Bus Element In2 : Inport  PortName=Desired Fuel
  Bus Element In3 : Inport  Port=2  PortName=Desired AFR
  Bus Element In1 : Inport  Port=3  PortName=Desired Air
  Bus Element Out1 : Outport  PortName=Final Air
  Bus Element Out2 : Outport  Port=2  PortName=Final Fuel
  Bus Element Out3 : Outport  Port=3  PortName=Final AFR

== system SystemComposer_Architecture/Controller/Core Functionality/Burner Control/Ignition Control ==
  Flame Detection : Subsystem
      settings: PortSchema="{\"entries\":[{\"content\":{\"headerSize\":26,\"margin\":15,\"minimumSpacing\":25,\"sides\":[{\"content\":{\"connectorIds\":[]},\"type\":\"ConnectorPlacement.EquallySpacedRectSide\",\"uuid\":\"096bda3c-cb26-41de-ada6-ed8c82f4dc3e\"},{\"content\":{\"connectorIds\":[],\"side\":\"RIGHT\"},\"type\":\"ConnectorPlacement.EquallySpacedRectSide\",\"uuid\":\"33a8afe9-c0b7-4d1e-b92f-6038b85d7ed2\"},{\"content\":{\"connectorIds\":[],\"side\":\"TOP\"},\"type\":\"ConnectorPlacement.EquallySpacedRectSide\",\"uuid\":\"f728da00-d767-486c-a498-31860175d68d\"}]},\"type\":\"ConnectorPlacement.EquallySpacedConnector\",\"uuid\":\"b1077154-7336-4249-93d2-0c64e27b627c\"}],\"packageUris\":[\"http://schema.mathworks.com/mf0/Connector/19700101\"],\"version\":\"1.0\"}"
  Ignitor Control : Subsystem
      settings: PortSchema="{\"entries\":[{\"content\":{\"headerSize\":26,\"margin\":15,\"minimumSpacing\":25,\"sides\":[{\"content\":{\"connectorIds\":[]},\"type\":\"ConnectorPlacement.EquallySpacedRectSide\",\"uuid\":\"096bda3c-cb26-41de-ada6-ed8c82f4dc3e\"},{\"content\":{\"connectorIds\":[],\"side\":\"RIGHT\"},\"type\":\"ConnectorPlacement.EquallySpacedRectSide\",\"uuid\":\"33a8afe9-c0b7-4d1e-b92f-6038b85d7ed2\"},{\"content\":{\"connectorIds\":[],\"side\":\"TOP\"},\"type\":\"ConnectorPlacement.EquallySpacedRectSide\",\"uuid\":\"f728da00-d767-486c-a498-31860175d68d\"}]},\"type\":\"ConnectorPlacement.EquallySpacedConnector\",\"uuid\":\"b1077154-7336-4249-93d2-0c64e27b627c\"}],\"packageUris\":[\"http://schema.mathworks.com/mf0/Connector/19700101\"],\"version\":\"1.0\"}"
  Bus Element Out1 : Outport  PortName=Flame Detected
  Bus Element Out2 : Outport  Port=2  PortName=Ignitiion Status

== system SystemComposer_Architecture/Controller/Core Functionality/Burner Control/Ignition Control/Flame Detection ==

== system SystemComposer_Architecture/Controller/Core Functionality/Burner Control/Ignition Control/Ignitor Control ==
